simulink model "model"  (R2019b)
settings: Solver=ode4  StartTime=0.0  StopTime=150.0  FixedStep=0.01  RelTol=1e-3
values from neighbouring files (symbols this model uses):
  A = 1.8    [Param.m]
  B = 0.0002    [Param.m]
  Cd = 0.3    [Param.m]
  G = 11    [Param.m]
  g = 9.81    [Param.m]
  J = 0.05    [Param.m]
  La_plus_Lfield = 6.008e-03    (= 0.006008)    [Param.m]
  Laf = 1.766e-03    (= 0.001766)    [Param.m]
  m = 800    [Param.m]
  r = 0.25    [Param.m]
  ro = 1.25    [Param.m]
  urr = 0.015    [Param.m]
libraries: simulink x1
settings Model: Creator=Łukasz  LastModifiedBy=Łukasz

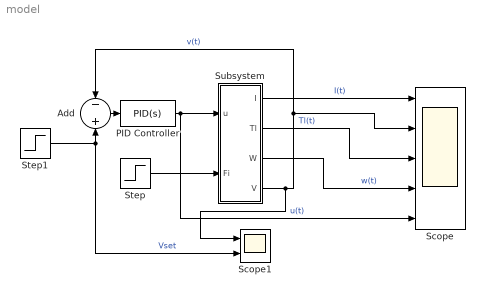
== system model ==
  Add : Sum  Inputs=-+
  PID Controller : simulink/Continuous/PID Controller  Controller=PID  Form=Parallel  TimeDomain=Continuous-time  SampleTime=-1  IntegratorMethod=Forward Euler  FilterMethod=Forward Euler  ControllerParametersSource=internal  P=52.2511943146378  I=69.1097396078928  D=-2.87080144544635  UseFilter=on  N=18.2009084597329  TunerSelectOption=Transfer Function Based (PID Tuner App)  InitialConditionSource=internal  InitialConditionForIntegrator=0  InitialConditionForFilter=0  DifferentiatorICPrevScaledInput=0  ExternalReset=none  TrackingMode=off  Kt=1  LimitOutput=on  UpperSaturationLimit=48  LowerSaturationLimit=0  LinearizeAsGain=on  AntiWindupMode=clamping  Kb=1  POutMin=[]  POutMax=[]  IOutMin=[]  IOutMax=[]  DOutMin=[]  DOutMax=[]  NOutMin=[]  NOutMax=[]  SumOutMin=[]  SumOutMax=[]  SaturationOutMin=[]  SaturationOutMax=[]  PParamMin=[]  PParamMax=[]  IParamMin=[]  IParamMax=[]  DParamMin=[]  DParamMax=[]  NParamMin=[]  NParamMax=[]  KbParamMin=[]  KbParamMax=[]  KtParamMin=[]  KtParamMax=[]  KbOutMin=[]  KbOutMax=[]  KtOutMin=[]  KtOutMax=[]  IntegratorOutMin=[]  IntegratorOutMax=[]  FilterOutMin=[]  FilterOutMax=[]  SumI1OutMin=[]  SumI1OutMax=[]  SumI2OutMin=[]  SumI2OutMax=[]  SumI3OutMin=[]  SumI3OutMax=[]  SumI4OutMin=[]  SumI4OutMax=[]  SumDOutMin=[]  SumDOutMax=[]  DifferentiatorOutMin=[]  DifferentiatorOutMax=[]  FilterDiffOutCoefMin=[]  FilterDiffOutCoefMax=[]  ReciprocalOutMin=[]  ReciprocalOutMax=[]  SumDenOutMin=[]  SumDenOutMax=[]  SumNumOutMin=[]  SumNumOutMax=[]  DivideOutMin=[]  DivideOutMax=[]  IntegratorContinuousStateAttributes=''  IntegratorStateMustResolveToSignalObject=off  IntegratorRTWStateStorageClass=Auto  FilterContinuousStateAttributes=''  FilterStateMustResolveToSignalObject=off  FilterRTWStateStorageClass=Auto  ParallelPVariant=InternalParameters  IdealPVariant=Disabled  IVariant=InternalParameters  DVariant=InternalParameters  IntegratorVariant=Continuous  SatVariant=Enabled  AWVariant=ContClampingParallel  PCopyVariant=Disabled  TRVariant=Disabled  FdbkBlocksVariant=Forward  IdealPFdbkVariant=Disabled  SatFdbkVariant=Disabled  DerivativeFilterVariant=ContFilter  NVariant=InternalParameters  NCopyVariant=Disabled  FilterICVariant=InternalICsFilter  IntegratorICVariant=InternalICs  ExternalResetVariant=Disabled  TRSumVariant=Passthrough  SumFdbkVariant=Disabled  SumVariant=Sum_PID
  Scope : Scope  NumInputPorts=5
  Scope1 : Scope  NumInputPorts=2
  Step : Step  Time=50  After=3  SampleTime=0
  Step1 : Step  After=10  SampleTime=0
  Subsystem : Subsystem
  wires:
  Subsystem/1(I) -> Scope/1  "I(t)"
  Subsystem/3(W) -> Scope/4  "w(t)"
  Subsystem/2(Tl) -> Scope/3  "Tl(t)"
  PID Controller/1 -> Scope/5, Subsystem/1(u)  "u(t)"
  Step/1 -> Subsystem/2(Fi)
  Add/1 -> PID Controller/1
  Step1/1 -> Scope1/2, Add/2  "Vset"
  Subsystem/4(V) -> Scope1/1, Add/1, Scope/2  "v(t)"

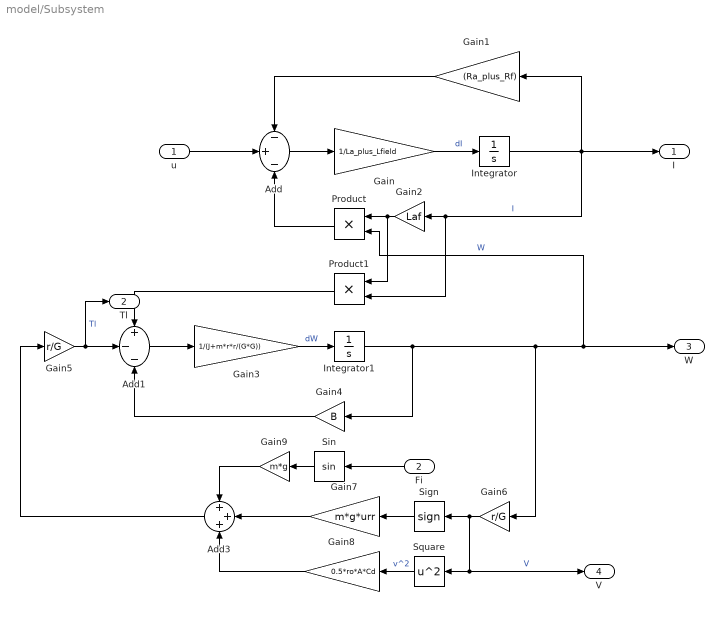
== system model/Subsystem ==
  u : Inport
  Fi : Inport  Port=2
  Add : Sum  Inputs=-+-
  Add1 : Sum  Inputs=+--
  Add3 : Sum  Inputs=+++
  Gain : Gain  Gain=1/La_plus_Lfield
  Gain1 : Gain  Gain=(Ra_plus_Rf)
  Gain2 : Gain  Gain=Laf
  Gain3 : Gain  Gain=1/(J+m*r*r/(G*G))
  Gain4 : Gain  Gain=B
  Gain5 : Gain  Gain=r/G
  Gain6 : Gain  Gain=r/G
  Gain7 : Gain  Gain=m*g*urr
  Gain8 : Gain  Gain=0.5*ro*A*Cd
  Gain9 : Gain  Gain=m*g
  Integrator : Integrator
  Integrator1 : Integrator
  Product : Product
  Product1 : Product
  Sign : Signum
  Sin : Trigonometry
  Square : Math  Operator=square  SignedPower=off  SaturateOnIntegerOverflow=on
  I : Outport
  Tl : Outport  Port=2
  W : Outport  Port=3
  V : Outport  Port=4
  wires:
  Fi/1 -> Sin/1
  Integrator1/1 -> Gain4/1, Gain6/1, W/1, Product/2  "W"
  Integrator/1 -> I/1, Product1/2, Gain2/1, Gain1/1  "I"
  Gain6/1 -> V/1, Square/1, Sign/1  "V"
  Gain/1 -> Integrator/1  "dI"
  Gain2/1 -> Product/1, Product1/1
  Gain1/1 -> Add/1
  Add/1 -> Gain/1
  Product/1 -> Add/3
  Gain4/1 -> Add1/3
  Gain9/1 -> Add3/1
  Gain3/1 -> Integrator1/1  "dW"
  Gain5/1 -> Tl/1, Add1/2  "Tl"
  Add1/1 -> Gain3/1
  Gain7/1 -> Add3/2
  Sign/1 -> Gain7/1
  Product1/1 -> Add1/1
  Add3/1 -> Gain5/1
  Square/1 -> Gain8/1  "v^2"
  Sin/1 -> Gain9/1
  Gain8/1 -> Add3/3
  u/1 -> Add/2
